simulink model "Altitude_Mode"  (Simulink 8.0)
settings: configuration reference "configSetObj_autopilot" (kept outside this file)
undefined symbols (not defined in the file): DiscIntNeverNeededParam
libraries: aerolibconvert2 x2, simulink x2
settings Model: Creator=bpotter  LastModifiedBy=ssauvage  CovSaveName=covdata_pitchAP  CovMetricSettings=dcmtre  CovHTMLOptions=-aTS=1 -bRG=1 -bTC=1 -hTR=1 -nFC=0 -scm=1 -bcm=1  CovCumulativeVarName=covCumulativeData_pitchAP  CovCumulativeReport=on  CovReportOnPause=off
settings ConfigSet: SourceLocation=Base Workspace

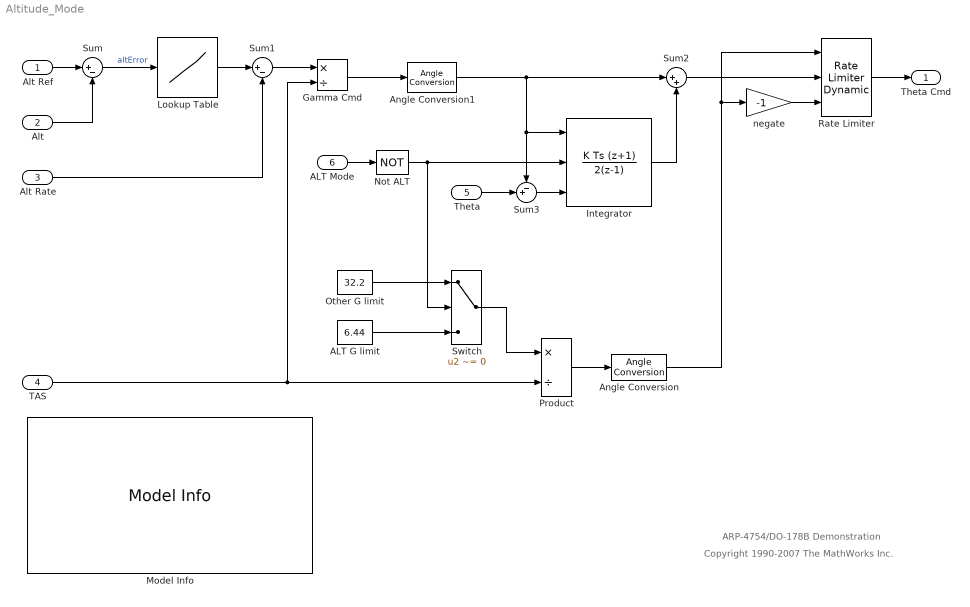
== system Altitude_Mode ==
  note: Copyright 1990-2007 The MathWorks Inc.
  note: ARP-4754/DO-178B Demonstration
  Alt Ref : Inport  OutDataTypeStr=double  PortDimensions=1  SampleTime=1/40  Interpolate=off
  Alt : Inport  Port=2  OutDataTypeStr=double  PortDimensions=1  SampleTime=1/40  Interpolate=off
  Alt Rate : Inport  Port=3  OutDataTypeStr=double  PortDimensions=1  SampleTime=1/40  Interpolate=off
  TAS : Inport  Port=4  OutDataTypeStr=double  PortDimensions=1  SampleTime=1/40  Interpolate=off
  Theta : Inport  Port=5  OutDataTypeStr=double  PortDimensions=1  SampleTime=1/40  Interpolate=off
  ALT Mode : Inport  Port=6  OutDataTypeStr=boolean  PortDimensions=1  SampleTime=1/40  Interpolate=off
  ALT G limit : Constant  Value=6.44  OutDataTypeStr=double
  Angle Conversion : aerolibconvert2/Angle Conversion  IU=rad  OU=deg
  Angle Conversion1 : aerolibconvert2/Angle Conversion  IU=rad  OU=deg
  Gamma Cmd : Product  Inputs=*/  RndMeth=Zero
  Integrator : DiscreteIntegrator  IntegratorMethod=Integration: Trapezoidal  gainval=0.2  ExternalReset=level  InitialConditionSource=external  InitialConditionMode=State only (most efficient)  SampleTime=1/40  LimitOutput=on  UpperSaturationLimit=20  LowerSaturationLimit=-20  IgnoreLimit=on  ICPrevOutput=DiscIntNeverNeededParam  ICPrevScaledInput=DiscIntNeverNeededParam
      settings: AttributesFormatString=K = %<gainval>\n%<LowerSaturationLimit> to %<UpperSaturationLimit> (deg)
  Lookup Table : Lookup  InputValues=[-544 -206 -116 -52 0 52 116 206]  Table=[-42 -26 -19 -13 0 13 19 26]  LookUpMeth=Interpolation-Use End Values
  Model Info : simulink/Model-Wide Utilities/Model Info  InitialBlockCM=None  BlockCM=None  Frame=on  DisplayStringWithTags=|  HorizontalTextAlignment=Left  LeftAlignmentValue=0.02  SourceBlockDiagram=Altitude_Mode  TagMaxNumber=20
      | Altitude Mode
      | Author: %<LastModifiedBy>
      | Version: %<ModelVersion>
      | Date: %<LastModificationDate>
      | DO-178B Software Lifecycle Data:
      |   11.9 Software Requirements Data
      |   11.10 Design Description
      | DO-178B Objectives:
      |   5.2.1a Low Level Requirements are Developed
      |   5.2.1a Software Architecture is Developed
      |   5.2.1b  Derived Low Level Requirements are Developed
  Not ALT : Logic  Operator=NOT  IconShape=distinctive  AllPortsSameDT=off  OutDataTypeStr=boolean
  Other G limit : Constant  Value=32.2  OutDataTypeStr=double
  Product : Product  Inputs=*/  RndMeth=Zero
  Rate Limiter : simulink/Discontinuities/Rate Limiter Dynamic
  Sum : Sum  Inputs=|+-
  Sum1 : Sum  Inputs=|+-
  Sum2 : Sum  Inputs=|++
  Sum3 : Sum  Inputs=-+|
  Switch : Switch  Criteria=u2 ~= 0
  negate : Gain  Gain=-1
  Theta Cmd : Outport  OutDataTypeStr=double  PortDimensions=1  SampleTime=1/40
  wires:
  Other G limit/1 -> Switch/1
  ALT G limit/1 -> Switch/3
  Switch/1 -> Product/1
  Theta/1 -> Sum3/2
  Sum3/1 -> Integrator/3
  Integrator/1 -> Sum2/2
  ALT Mode/1 -> Not ALT/1
  Not ALT/1 -> Switch/2, Integrator/2
  Angle Conversion1/1 -> Sum3/1, Integrator/1, Sum2/1
  Angle Conversion/1 -> negate/1, Rate Limiter/1
  Product/1 -> Angle Conversion/1
  Sum2/1 -> Rate Limiter/2
  Gamma Cmd/1 -> Angle Conversion1/1
  negate/1 -> Rate Limiter/3
  Sum1/1 -> Gamma Cmd/1
  Lookup Table/1 -> Sum1/1
  Rate Limiter/1 -> Theta Cmd/1
  Sum/1 -> Lookup Table/1  "altError"
  Alt Ref/1 -> Sum/1
  TAS/1 -> Gamma Cmd/2, Product/2
  Alt Rate/1 -> Sum1/2
  Alt/1 -> Sum/2
